simulink model "ESTS_TFX_test"  (R2023b)
settings: Solver=VariableStepAuto  StartTime=0.0  StopTime=10.0  RelTol=1e-3
libraries: ESTS_TFX x1
settings Model: Creator=blatak  LastModifiedBy=blatak

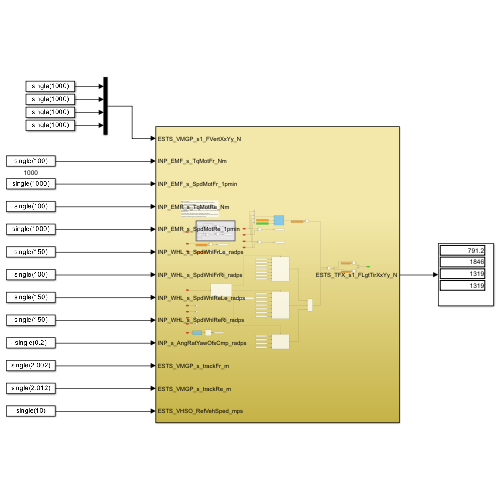
[thumbnail: Simulink's stored preview of the top-level diagram]
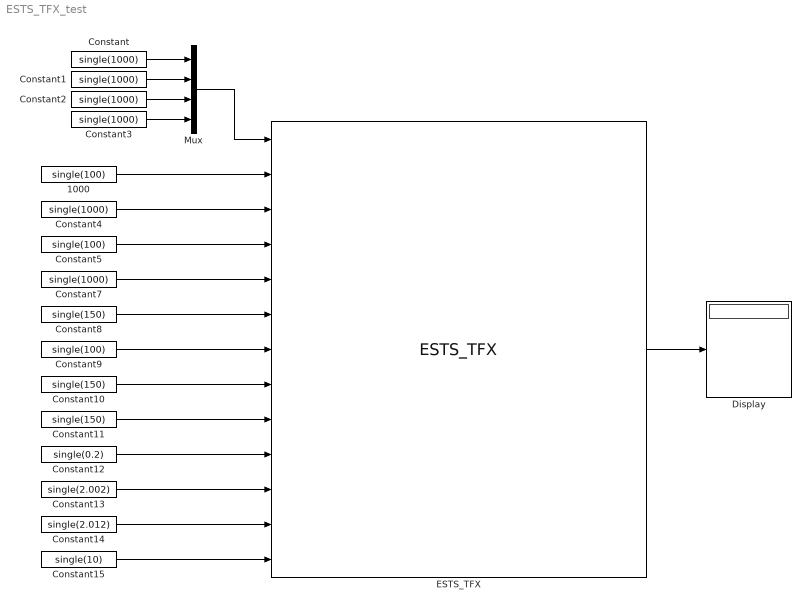
== system ESTS_TFX_test ==
  1000 : Constant  Value=single(100)
  Constant{,1..4,7} (6 alike) : Constant  Value=single(1000)
  Constant10 : Constant  Value=single(150)
  Constant11 : Constant  Value=single(150)
  Constant12 : Constant  Value=single(0.2)
  Constant13 : Constant  Value=single(2.002)
  Constant14 : Constant  Value=single(2.012)
  Constant15 : Constant  Value=single(10)
  Constant5 : Constant  Value=single(100)
  Constant8 : Constant  Value=single(150)
  Constant9 : Constant  Value=single(100)
  Display : Display
  ESTS_TFX : ESTS_TFX/ESTS_TFX  SystemSampleTime=-1  VariantActivationTime=update diagram  AllowFlexibleInterface=on  Latency=0  AutoFrameSizeCalculation=off
      link override 1-D Lookup Table: BreakpointsForDimension1=ESTS_TFX_p1_SpdRefVehXLim_kmph  Table=ESTS_TFX_p1_SpdWhlDifLim_radps
      link override If Action Subsystem/If Action Subsystem3/1-D Lookup Table: BreakpointsForDimension1=ESTS_TFX_p1_TqWhlFrX_Nm  Table=ESTS_TFX_py_TqWhlDifFr_Nm
  Mux : Mux
  wires:
  Constant/1 -> Mux/1
  Constant1/1 -> Mux/2
  Constant2/1 -> Mux/3
  Constant3/1 -> Mux/4
  Mux/1 -> ESTS_TFX/1
  Constant5/1 -> ESTS_TFX/4
  Constant4/1 -> ESTS_TFX/3
  1000/1 -> ESTS_TFX/2
  Constant7/1 -> ESTS_TFX/5
  Constant8/1 -> ESTS_TFX/6
  Constant9/1 -> ESTS_TFX/7
  Constant10/1 -> ESTS_TFX/8
  Constant11/1 -> ESTS_TFX/9
  Constant12/1 -> ESTS_TFX/10
  Constant13/1 -> ESTS_TFX/11
  Constant14/1 -> ESTS_TFX/12
  Constant15/1 -> ESTS_TFX/13
  ESTS_TFX/1 -> Display/1
